simulink model "Simulador_CIC2021_Matlab2021a"  (R2021a)
settings: Solver=FixedStepAuto  StartTime=0.0  StopTime=inf  FixedStep=Ts  MaxStep=Ts  RelTol=1e-3
InitFcn:
  | Ts_com =0.0200;
  | Ts= 0.0100;
  | load DatosCref;
StopFcn:
  | clear tf Ts Ts_com tout DatosCrefC1 DatosCrefC2;
undefined symbols (not defined in the file): sigbuilder_block, Ts3
settings Model: Creator=jarico  LastModifiedBy=javier
settings SolverCC: ZeroCrossControl=DisableAll  AlgebraicLoopSolver=TrustRegion
settings DataIOCC: SaveFormat=StructureWithTime  SignalLogging=off  DSMLogging=off  ReturnWorkspaceOutputs=off
settings DebuggingCC: SFMachineParentedDataDiag=warning  ArithmeticOperatorsInVariantConditions=warning
settings SFSimCC: CustomCodeUndefinedFunction=UseInterfaceOnly

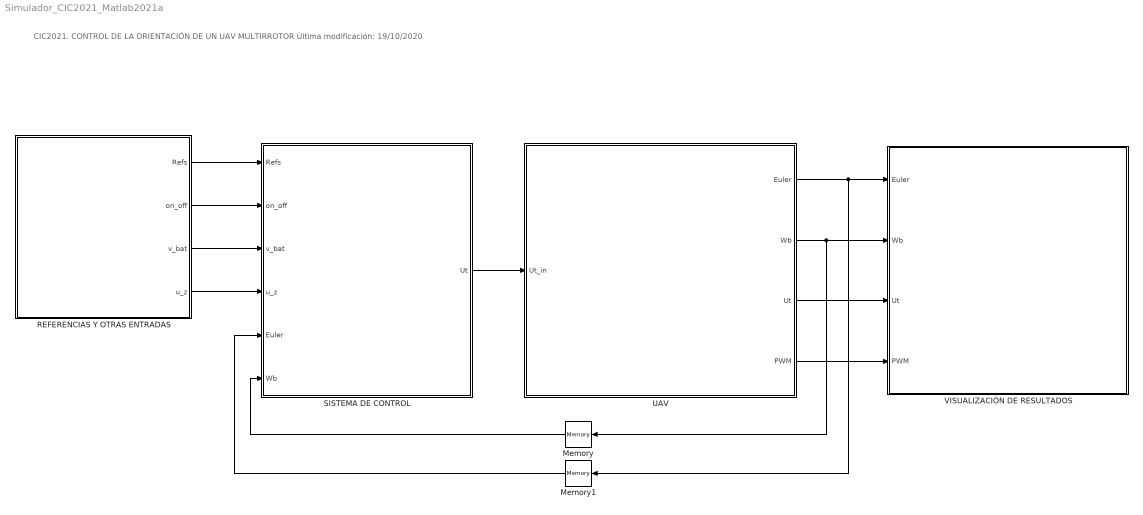
== system Simulador_CIC2021_Matlab2021a ==
  note: CIC2021. CONTROL DE LA ORIENTACIÓN DE UN UAV MULTIRROTOR
      |
      | Última modificación: 19/10/2020
  Memory : Memory
  Memory1 : Memory
  REFERENCIAS Y OTRAS ENTRADAS : Subsystem
  SISTEMA DE CONTROL : Subsystem
  UAV : Subsystem  SystemSampleTime=Ts3  mask(CONCURSO DE INGENIERÍA DE CONTROL CIC2021){Categoria=Categoría 1}
      mask prompts: Categoria "Seleccione categoría:"
      mask help: Modelo dinámico del UAV
      mask TypeOptions Categoria: Categoría 1 | Categoría 2
      mask DialogControl Container7 Prompt: Operación del sistema
      mask Display: image(imread('UAV.png'));
  VISUALIZACIÓN DE RESULTADOS : Subsystem
  wires:
  UAV/4(PWM) -> VISUALIZACIÓN DE RESULTADOS/4(PWM)
  UAV/3(Ut) -> VISUALIZACIÓN DE RESULTADOS/3(Ut)
  REFERENCIAS Y OTRAS ENTRADAS/1(Refs) -> SISTEMA DE CONTROL/1(Refs)
  REFERENCIAS Y OTRAS ENTRADAS/2(on_off) -> SISTEMA DE CONTROL/2(on_off)
  REFERENCIAS Y OTRAS ENTRADAS/3(v_bat) -> SISTEMA DE CONTROL/3(v_bat)
  REFERENCIAS Y OTRAS ENTRADAS/4(u_z) -> SISTEMA DE CONTROL/4(u_z)
  SISTEMA DE CONTROL/1(Ut) -> UAV/1(Ut_in)
  UAV/2(Wb) -> Memory/1, VISUALIZACIÓN DE RESULTADOS/2(Wb)
  UAV/1(Euler) -> Memory1/1, VISUALIZACIÓN DE RESULTADOS/1(Euler)
  Memory/1 -> SISTEMA DE CONTROL/6(Wb)
  Memory1/1 -> SISTEMA DE CONTROL/5(Euler)

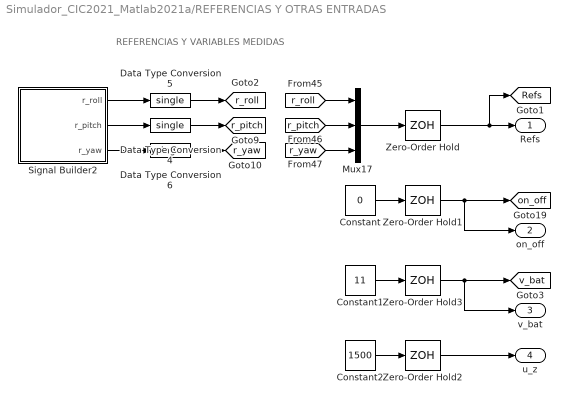
== system Simulador_CIC2021_Matlab2021a/REFERENCIAS Y OTRAS ENTRADAS ==
  note: REFERENCIAS Y VARIABLES MEDIDAS
  Constant : Constant  Value=0  OutDataTypeStr=int16
  Constant1 : Constant  Value=11  OutDataTypeStr=single
  Constant2 : Constant  Value=1500  OutDataTypeStr=single
  Data Type Conversion4 : DataTypeConversion  OutDataTypeStr=single
  Data Type Conversion5 : DataTypeConversion  OutDataTypeStr=single
  Data Type Conversion6 : DataTypeConversion  OutDataTypeStr=single
  Mux17 : Mux  Inputs=3
  Signal Builder2 : Subsystem  Tag=STV Subsys  LoadFcn=sigbuilder_block('load');  StartFcn=sigbuilder_block('start');  StopFcn=sigbuilder_block('stop');  ClipboardFcn=sigbuilder_block('clipboard');  mask(Sigbuilder block){tuvar=[0:10]}
      mask help: Simulink:masks:SigbuilderBlock_MD
      mask init:
      | if ~strcmp(get_param(bdroot(gcbh),'SimulationStatus'),'stopped') tuvar = sigbuilder_block('maskInit'); end
      settings: CopyFcn=sigbuilder_block('copy');  DeleteFcn=sigbuilder_block('delete');  ModelCloseFcn=sigbuilder_block('modelClose');  PreSaveFcn=sigbuilder_block('preSave');  PauseFcn=sigbuilder_block('pause');  ContinueFcn=sigbuilder_block('continue');  NameChangeFcn=sigbuilder_block('namechange');  OpenFcn=sigbuilder_block('open',[571.8 30.6 574.8 516.6 ]);  CloseFcn=sigbuilder_block('close');
      mask Display: plot(0, 0, 100, 100,[2, 2, 32, 32, 2], [68, 8, 8, 68, 68],[32, 2], [38, 38], [32, 19, 2],[53, 60, 44], [32, 17, 17, 2],[16, 16, 31, 31]);txt = getActiveGroup(gcbh);text(2, 100, txt,'verticalAlignment', 'top');
  Zero-Order Hold : ZeroOrderHold  SampleTime=Ts_com
  Zero-Order Hold1 : ZeroOrderHold  SampleTime=Ts_com
  Zero-Order Hold2 : ZeroOrderHold  SampleTime=Ts_com
  Zero-Order Hold3 : ZeroOrderHold  SampleTime=Ts
  Refs : Outport  VectorParamsAs1DForOutWhenUnconnected=off
  on_off : Outport  Port=2  VectorParamsAs1DForOutWhenUnconnected=off
  v_bat : Outport  Port=3  VectorParamsAs1DForOutWhenUnconnected=off
  u_z : Outport  Port=4  VectorParamsAs1DForOutWhenUnconnected=off
  tag scope: Refs=global, on_off=global, r_pitch=global, r_roll=global, r_yaw=global, v_bat=global
  wires:
  Constant/1 -> Zero-Order Hold1/1
  Mux17/1 -> Zero-Order Hold/1
  [r_roll] -> Mux17/1
  Data Type Conversion5/1 -> [r_roll]
  Data Type Conversion6/1 -> [r_yaw]
  [r_pitch] -> Mux17/2
  Data Type Conversion4/1 -> [r_pitch]
  [r_yaw] -> Mux17/3
  Signal Builder2/3(r_yaw) -> Data Type Conversion6/1
  Signal Builder2/2(r_pitch) -> Data Type Conversion4/1
  Signal Builder2/1(r_roll) -> Data Type Conversion5/1
  Constant1/1 -> Zero-Order Hold3/1
  Constant2/1 -> Zero-Order Hold2/1
  Zero-Order Hold/1 -> [Refs], Refs/1
  Zero-Order Hold1/1 -> on_off/1, [on_off]
  Zero-Order Hold2/1 -> u_z/1
  Zero-Order Hold3/1 -> [v_bat], v_bat/1

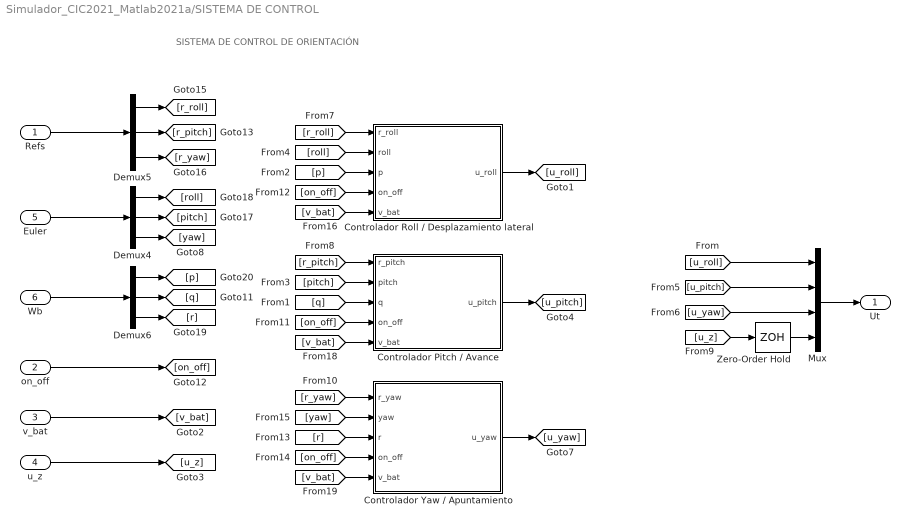
== system Simulador_CIC2021_Matlab2021a/SISTEMA DE CONTROL ==
  note: SISTEMA DE CONTROL DE ORIENTACIÓN
  Refs : Inport
  on_off : Inport  Port=2
  v_bat : Inport  Port=3
  u_z : Inport  Port=4
  Euler : Inport  Port=5
  Wb : Inport  Port=6
  Controlador Pitch / Avance : Subsystem
  Controlador Roll / Desplazamiento lateral : Subsystem
  Controlador Yaw / Apuntamiento : Subsystem
  Demux4 : Demux  Outputs=3
  Demux5 : Demux  Outputs=3
  Demux6 : Demux  Outputs=3
  Mux : Mux
  Zero-Order Hold : ZeroOrderHold  SampleTime=Ts
  Ut : Outport  VectorParamsAs1DForOutWhenUnconnected=off
  wires:
  [p] -> Controlador Roll / Desplazamiento lateral/3(p)
  [roll] -> Controlador Roll / Desplazamiento lateral/2(roll)
  [r_roll] -> Controlador Roll / Desplazamiento lateral/1(r_roll)
  Controlador Pitch / Avance/1(u_pitch) -> [u_pitch]
  Controlador Roll / Desplazamiento lateral/1(u_roll) -> [u_roll]
  [on_off] -> Controlador Roll / Desplazamiento lateral/4(on_off)
  [r_pitch] -> Controlador Pitch / Avance/1(r_pitch)
  [pitch] -> Controlador Pitch / Avance/2(pitch)
  [q] -> Controlador Pitch / Avance/3(q)
  [on_off] -> Controlador Pitch / Avance/4(on_off)
  [u_roll] -> Mux/1
  [u_pitch] -> Mux/2
  [u_yaw] -> Mux/3
  [u_z] -> Zero-Order Hold/1
  Mux/1 -> Ut/1
  Demux5/1 -> [r_roll]
  Demux4/2 -> [pitch]
  Demux4/3 -> [yaw]
  Demux5/2 -> [r_pitch]
  Demux5/3 -> [r_yaw]
  Demux4/1 -> [roll]
  Demux6/2 -> [q]
  Wb/1 -> Demux6/1
  Demux6/1 -> [p]
  Refs/1 -> Demux5/1
  on_off/1 -> [on_off]
  Euler/1 -> Demux4/1
  Demux6/3 -> [r]
  u_z/1 -> [u_z]
  v_bat/1 -> [v_bat]
  [yaw] -> Controlador Yaw / Apuntamiento/2(yaw)
  Controlador Yaw / Apuntamiento/1(u_yaw) -> [u_yaw]
  [on_off] -> Controlador Yaw / Apuntamiento/4(on_off)
  [r] -> Controlador Yaw / Apuntamiento/3(r)
  [r_yaw] -> Controlador Yaw / Apuntamiento/1(r_yaw)
  [v_bat] -> Controlador Roll / Desplazamiento lateral/5(v_bat)
  [v_bat] -> Controlador Pitch / Avance/5(v_bat)
  [v_bat] -> Controlador Yaw / Apuntamiento/5(v_bat)
  Zero-Order Hold/1 -> Mux/4

== system Simulador_CIC2021_Matlab2021a/UAV ==
  Ut_in : Inport
  " UAV" : Subsystem
      mask help: Simulink:masks:GenSFuncDesc_MD
      mask Help: eval('feval(''rtwprivate'',''rtwhelpview'',''rtw_sfcn_block'')');
  Constant : Constant  Value=Categoria
  Data Type Conversion : DataTypeConversion  OutDataTypeStr=single
  Demux : Demux
  Euler : Outport  VectorParamsAs1DForOutWhenUnconnected=off
  Wb : Outport  Port=2  VectorParamsAs1DForOutWhenUnconnected=off
  Ut : Outport  Port=3  VectorParamsAs1DForOutWhenUnconnected=off
  PWM : Outport  Port=4  VectorParamsAs1DForOutWhenUnconnected=off
  tag scope: Categoria=global
  wires:
  Demux/4 -> " UAV"/4(u_z)
  [v_bat] -> " UAV"/5(v_bat)
  Constant/1 -> Data Type Conversion/1
  " UAV"/3(Ut) -> Ut/1
  " UAV"/4(PWM) -> PWM/1
  " UAV"/1(Euler) -> Euler/1
  " UAV"/2(Wb) -> Wb/1
  Demux/3 -> " UAV"/3(u_yaw)
  Demux/2 -> " UAV"/2(u_pitch)
  Demux/1 -> " UAV"/1(u_roll)
  Ut_in/1 -> Demux/1
  Data Type Conversion/1 -> " UAV"/6(Categoria), [Categoria]

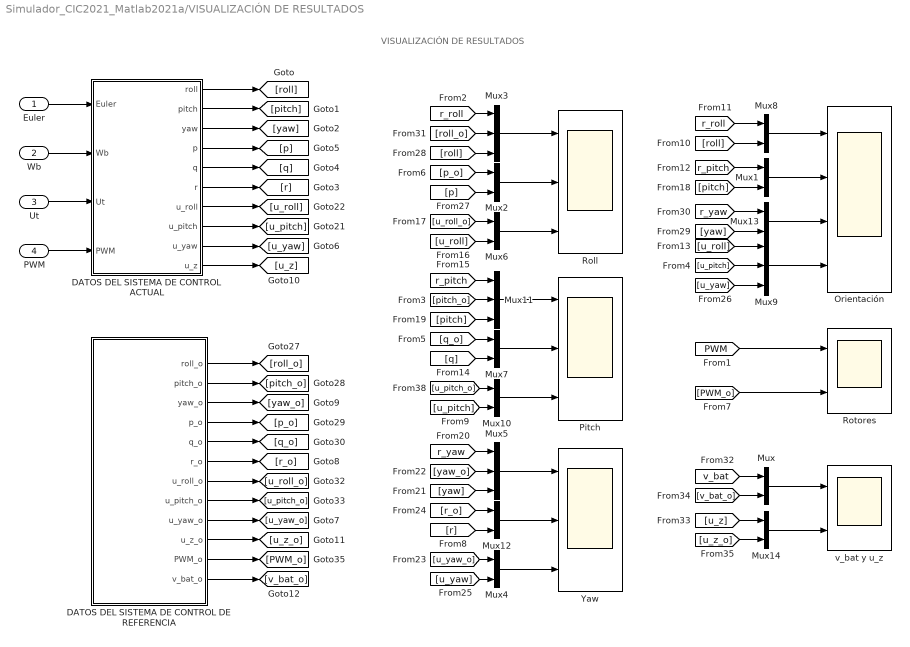
== system Simulador_CIC2021_Matlab2021a/VISUALIZACIÓN DE RESULTADOS ==
  note: VISUALIZACIÓN DE RESULTADOS
  Euler : Inport
  Wb : Inport  Port=2
  Ut : Inport  Port=3
  PWM : Inport  Port=4
  DATOS DEL SISTEMA DE CONTROL ACTUAL : Subsystem
  DATOS DEL SISTEMA DE CONTROL DE REFERENCIA : Subsystem
  Mux{,1..2,4,6..8,10,12..14} (11 alike) : Mux  Inputs=2
  Mux{3,5,9,11} (4 alike) : Mux  Inputs=3
  Orientación : Scope  NumInputPorts=4
  Pitch : Scope  NumInputPorts=3
  Roll : Scope  NumInputPorts=3
  Rotores : Scope  NumInputPorts=2
  Yaw : Scope  NumInputPorts=3
  v_bat y u_z : Scope  NumInputPorts=2
  wires:
  DATOS DEL SISTEMA DE CONTROL DE REFERENCIA/9(u_yaw_o) -> [u_yaw_o]
  DATOS DEL SISTEMA DE CONTROL DE REFERENCIA/6(r_o) -> [r_o]
  DATOS DEL SISTEMA DE CONTROL DE REFERENCIA/3(yaw_o) -> [yaw_o]
  DATOS DEL SISTEMA DE CONTROL ACTUAL/9(u_yaw) -> [u_yaw]
  DATOS DEL SISTEMA DE CONTROL ACTUAL/6(r) -> [r]
  DATOS DEL SISTEMA DE CONTROL ACTUAL/3(yaw) -> [yaw]
  [yaw] -> Mux13/2
  [r_yaw] -> Mux13/1
  Mux13/1 -> Orientación/3
  [u_yaw] -> Mux9/3
  [r_o] -> Mux12/1
  [u_yaw_o] -> Mux4/1
  [yaw] -> Mux5/3
  [yaw_o] -> Mux5/2
  [u_yaw] -> Mux4/2
  [r] -> Mux12/2
  [r_yaw] -> Mux5/1
  Mux4/1 -> Yaw/3
  Mux12/1 -> Yaw/2
  Mux5/1 -> Yaw/1
  Mux11/1 -> Pitch/1
  Mux7/1 -> Pitch/2
  Mux10/1 -> Pitch/3
  [r_pitch] -> Mux11/1
  [q] -> Mux7/2
  [u_pitch] -> Mux10/2
  Mux6/1 -> Roll/3
  Mux2/1 -> Roll/2
  [u_roll] -> Mux6/2
  [p] -> Mux2/2
  PWM/1 -> DATOS DEL SISTEMA DE CONTROL ACTUAL/4(PWM)
  DATOS DEL SISTEMA DE CONTROL ACTUAL/8(u_pitch) -> [u_pitch]
  DATOS DEL SISTEMA DE CONTROL ACTUAL/7(u_roll) -> [u_roll]
  DATOS DEL SISTEMA DE CONTROL ACTUAL/5(q) -> [q]
  DATOS DEL SISTEMA DE CONTROL ACTUAL/4(p) -> [p]
  DATOS DEL SISTEMA DE CONTROL ACTUAL/2(pitch) -> [pitch]
  DATOS DEL SISTEMA DE CONTROL ACTUAL/1(roll) -> [roll]
  Ut/1 -> DATOS DEL SISTEMA DE CONTROL ACTUAL/3(Ut)
  Wb/1 -> DATOS DEL SISTEMA DE CONTROL ACTUAL/2(Wb)
  Euler/1 -> DATOS DEL SISTEMA DE CONTROL ACTUAL/1(Euler)
  DATOS DEL SISTEMA DE CONTROL DE REFERENCIA/4(p_o) -> [p_o]
  DATOS DEL SISTEMA DE CONTROL DE REFERENCIA/5(q_o) -> [q_o]
  DATOS DEL SISTEMA DE CONTROL DE REFERENCIA/11(PWM_o) -> [PWM_o]
  DATOS DEL SISTEMA DE CONTROL DE REFERENCIA/7(u_roll_o) -> [u_roll_o]
  DATOS DEL SISTEMA DE CONTROL DE REFERENCIA/8(u_pitch_o) -> [u_pitch_o]
  DATOS DEL SISTEMA DE CONTROL DE REFERENCIA/1(roll_o) -> [roll_o]
  DATOS DEL SISTEMA DE CONTROL DE REFERENCIA/2(pitch_o) -> [pitch_o]
  [PWM] -> Rotores/1
  [pitch_o] -> Mux11/2
  [pitch] -> Mux11/3
  [r_roll] -> Mux3/1
  Mux9/1 -> Orientación/4
  [u_pitch_o] -> Mux10/1
  [q_o] -> Mux7/1
  [p_o] -> Mux2/1
  [u_roll_o] -> Mux6/1
  Mux3/1 -> Roll/1
  Mux1/1 -> Orientación/2
  [u_pitch] -> Mux9/2
  [u_roll] -> Mux9/1
  [pitch] -> Mux1/2
  [r_pitch] -> Mux1/1
  Mux8/1 -> Orientación/1
  [r_roll] -> Mux8/1
  [roll] -> Mux8/2
  [roll_o] -> Mux3/2
  [roll] -> Mux3/3
  [PWM_o] -> Rotores/2
  DATOS DEL SISTEMA DE CONTROL ACTUAL/10(u_z) -> [u_z]
  [v_bat] -> Mux/1
  [u_z] -> Mux14/1
  DATOS DEL SISTEMA DE CONTROL DE REFERENCIA/10(u_z_o) -> [u_z_o]
  DATOS DEL SISTEMA DE CONTROL DE REFERENCIA/12(v_bat_o) -> [v_bat_o]
  [v_bat_o] -> Mux/2
  [u_z_o] -> Mux14/2
  Mux/1 -> v_bat y u_z/1
  Mux14/1 -> v_bat y u_z/2

== system Simulador_CIC2021_Matlab2021a/REFERENCIAS Y OTRAS ENTRADAS/Signal Builder2 ==
  Demux : Demux  Tag=STV Demux  Outputs=3
      settings: DisplayOption=none
  FromWs : FromWorkspace  Tag=STV FromWs  VariableName=tuvar
      SigBuilderData=|
      | common.afterFinalStr = 'Extrapolate'
      | common.sampleTime = 0
      | dataSet.timeRange = [0 65]
      | dataSet.name = 'Group 1'
      | sbobj.Groups.Name = 'Group 1'
      | sbobj.Groups.Signals(1).Name = 'r_roll'
      | sbobj.Groups.Signals(1).XData = [0 5 5 10 10 25 25 30 30 40 40 65]
      | sbobj.Groups.Signals(1).YData = [0 0 200 200 0 0 -200 -200 200 200 0 0]
      | sbobj.Groups.Signals(2).Name = 'r_pitch'
      | sbobj.Groups.Signals(2).XData = [0 15 15 20 20 25 25 35 35 65]
      | sbobj.Groups.Signals(2).YData = [0 0 200 200 0 0 -200 -200 0 0]
      | sbobj.Groups.Signals(3).Name = 'r_yaw'
      | sbobj.Groups.Signals(3).XData = [0 45.3 50 55 60 65]
      | sbobj.Groups.Signals(3).YData = [0 0 -500 -500 0 0]
      | sbobj.Groups.TimeRange = [0 65]
  r_roll : Outport  Tag=STV Outport  VectorParamsAs1DForOutWhenUnconnected=off
  r_pitch : Outport  Tag=STV Outport  Port=2  VectorParamsAs1DForOutWhenUnconnected=off
  r_yaw : Outport  Tag=STV Outport  Port=3  VectorParamsAs1DForOutWhenUnconnected=off
  wires:
  Demux/3 -> r_yaw/1
  Demux/2 -> r_pitch/1
  FromWs/1 -> Demux/1
  Demux/1 -> r_roll/1

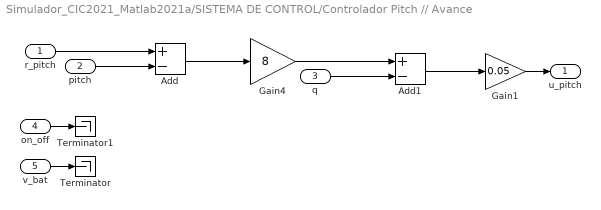
== system Simulador_CIC2021_Matlab2021a/SISTEMA DE CONTROL/Controlador Pitch // Avance ==
  r_pitch : Inport
  pitch : Inport  Port=2
  q : Inport  Port=3
  on_off : Inport  Port=4
  v_bat : Inport  Port=5
  Add : Sum  Inputs=+-
  Add1 : Sum  Inputs=+-
  Gain1 : Gain  Gain=0.05  OutDataTypeStr=single
  Gain4 : Gain  Gain=8
  Terminator : Terminator
  Terminator1 : Terminator
  u_pitch : Outport  VectorParamsAs1DForOutWhenUnconnected=off
  wires:
  Gain4/1 -> Add1/1
  r_pitch/1 -> Add/1
  Add/1 -> Gain4/1
  Add1/1 -> Gain1/1
  Gain1/1 -> u_pitch/1
  v_bat/1 -> Terminator/1
  on_off/1 -> Terminator1/1
  pitch/1 -> Add/2
  q/1 -> Add1/2

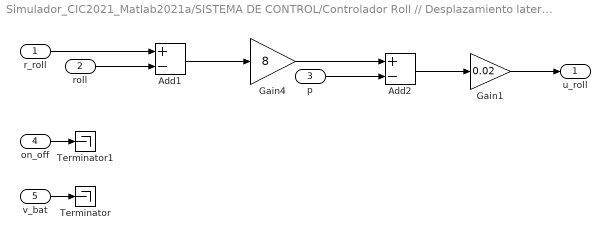
== system Simulador_CIC2021_Matlab2021a/SISTEMA DE CONTROL/Controlador Roll // Desplazamiento lateral ==
  r_roll : Inport
  roll : Inport  Port=2
  p : Inport  Port=3
  on_off : Inport  Port=4
  v_bat : Inport  Port=5
  Add1 : Sum  Inputs=+-
  Add2 : Sum  Inputs=+-
  Gain1 : Gain  Gain=0.02  OutDataTypeStr=single
  Gain4 : Gain  Gain=8
  Terminator : Terminator
  Terminator1 : Terminator
  u_roll : Outport  VectorParamsAs1DForOutWhenUnconnected=off
  wires:
  Gain1/1 -> u_roll/1
  v_bat/1 -> Terminator/1
  Gain4/1 -> Add2/1
  Add2/1 -> Gain1/1
  on_off/1 -> Terminator1/1
  Add1/1 -> Gain4/1
  r_roll/1 -> Add1/1
  roll/1 -> Add1/2
  p/1 -> Add2/2

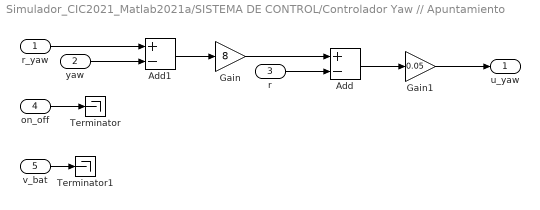
== system Simulador_CIC2021_Matlab2021a/SISTEMA DE CONTROL/Controlador Yaw // Apuntamiento ==
  r_yaw : Inport
  yaw : Inport  Port=2
  r : Inport  Port=3
  on_off : Inport  Port=4
  v_bat : Inport  Port=5
  Add : Sum  Inputs=+-
  Add1 : Sum  Inputs=+-
  Gain : Gain  Gain=8
  Gain1 : Gain  Gain=0.05
  Terminator : Terminator
  Terminator1 : Terminator
  u_yaw : Outport  VectorParamsAs1DForOutWhenUnconnected=off
  wires:
  r_yaw/1 -> Add1/1
  Add/1 -> Gain1/1
  Gain/1 -> Add/1
  r/1 -> Add/2
  yaw/1 -> Add1/2
  on_off/1 -> Terminator/1
  Add1/1 -> Gain/1
  Gain1/1 -> u_yaw/1
  v_bat/1 -> Terminator1/1

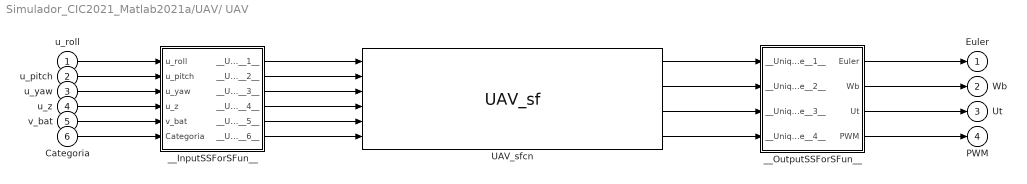
== system Simulador_CIC2021_Matlab2021a/UAV/ UAV ==
  u_roll : Inport
  u_pitch : Inport  Port=2
  u_yaw : Inport  Port=3
  u_z : Inport  Port=4
  v_bat : Inport  Port=5
  Categoria : Inport  Port=6
  " UAV_sfcn" : S-Function  FunctionName=UAV_sf  SFunctionModules=""  SFunctionDeploymentMode=off  EnableBusSupport=off  SFcnStateName=DWORK0  mask{rtw_sf_name=UAV_sf, showVar=off}
      mask prompts: rtw_sf_name "Simulink:masks:GenSFuncName_MP"; showVar "Simulink:masks:GenSFuncShowModuleList_MP"
      mask help: Simulink:masks:GenSFuncDesc_MD
      mask init:
      | displist = '';
      | if ~strcmp(get_param(gcb, 'FunctionName'), rtw_sf_name);
      |   set_param(gcb, 'FunctionName', rtw_sf_name);
      | end
      | % Check if we are generating code
      | rtw_mode = false;
      | if strcmpi(get_param(bdroot(gcb),'SimulationStatus'),'Initializing')
      | 	rtw_mode = strcmpi(get_param(bdroot(gcb),'BuildingRTWCode'),'on') && ...
      | 		~strcmpi(get_param(bdroot(gcb),'TargetStyle'),'SimulationTarget');
      | end
      | if showVar || rtw_mode
      | 	if exist('rtwsfunc') == 2 | exist('rtwsfunc') == 6
      | 		tmplist = rtwsfunc(rtw_sf_name,gcb);
      | 		tmplist = DAStudio.message('Simulink:masks:GenSFuncListOfModules_IC', tmplist);
      | 	elseif showVar
      | 		tmplist1 = DAStudio.message('Simulink:masks:GenSFuncListOfModules_IC', '');
      |         tmplist2 = DAStudio.message('Simulink:masks:GenSFuncNotLicensed_IC');
      |         tmplist = [tmplist1 tmplist2];
      |  	end
      | end
      | if showVar
      |   displist = tmplist;
      | end
      settings: SFcnIsStateOwnerBlock=on
      settings: CopyFcn=|
      | if ~strcmp(get_param(gcb,'Linkstatus'),'none') && ...
      | ~strcmp(get_param(gcb,'Linkstatus'),'implicit')
      |   set_param(gcb,'LinkStatus','none');
      | end
      mask Help: eval('feval(''rtwprivate'',''rtwhelpview'',''rtw_sfcn_block'')');
      mask Display:
      | port_label('input',1,'u_roll');
      | port_label('input',2,'u_pitch');
      | port_label('input',3,'u_yaw');
      | port_label('input',4,'u_z');
      | port_label('input',5,'v_bat');
      | port_label('input',6,'Categoria');
      | port_label('output',1,'Euler');
      | port_label('output',2,'Wb');
      | port_label('output',3,'Ut');
      | port_label('output',4,'PWM');
  __InputSSForSFun__ : Subsystem
  __OutputSSForSFun__ : Subsystem
  Euler : Outport  VectorParamsAs1DForOutWhenUnconnected=off
  Wb : Outport  Port=2  VectorParamsAs1DForOutWhenUnconnected=off
  Ut : Outport  Port=3  VectorParamsAs1DForOutWhenUnconnected=off
  PWM : Outport  Port=4  VectorParamsAs1DForOutWhenUnconnected=off
  wires:
  u_roll/1 -> __InputSSForSFun__/1(u_roll)
  u_pitch/1 -> __InputSSForSFun__/2(u_pitch)
  u_yaw/1 -> __InputSSForSFun__/3(u_yaw)
  u_z/1 -> __InputSSForSFun__/4(u_z)
  v_bat/1 -> __InputSSForSFun__/5(v_bat)
  Categoria/1 -> __InputSSForSFun__/6(Categoria)
  __InputSSForSFun__/1(__UniqueOutportName__1__) -> " UAV_sfcn"/1
  __InputSSForSFun__/2(__UniqueOutportName__2__) -> " UAV_sfcn"/2
  __InputSSForSFun__/3(__UniqueOutportName__3__) -> " UAV_sfcn"/3
  __InputSSForSFun__/4(__UniqueOutportName__4__) -> " UAV_sfcn"/4
  __InputSSForSFun__/5(__UniqueOutportName__5__) -> " UAV_sfcn"/5
  __InputSSForSFun__/6(__UniqueOutportName__6__) -> " UAV_sfcn"/6
  " UAV_sfcn"/1 -> __OutputSSForSFun__/1(__UniqueInportName__1__)
  " UAV_sfcn"/2 -> __OutputSSForSFun__/2(__UniqueInportName__2__)
  " UAV_sfcn"/3 -> __OutputSSForSFun__/3(__UniqueInportName__3__)
  " UAV_sfcn"/4 -> __OutputSSForSFun__/4(__UniqueInportName__4__)
  __OutputSSForSFun__/1(Euler) -> Euler/1
  __OutputSSForSFun__/2(Wb) -> Wb/1
  __OutputSSForSFun__/3(Ut) -> Ut/1
  __OutputSSForSFun__/4(PWM) -> PWM/1

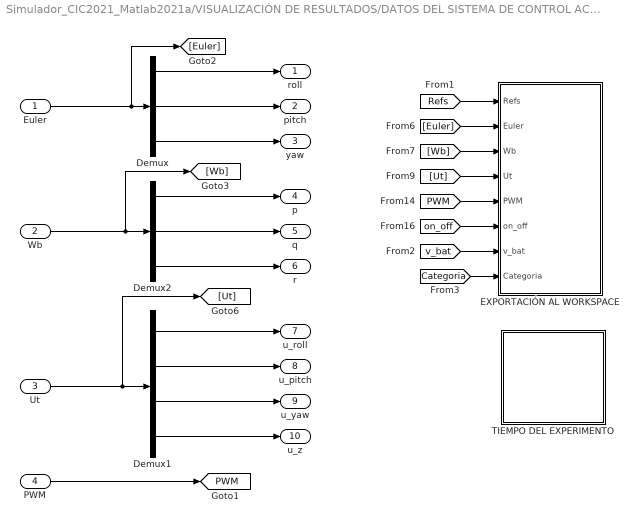
== system Simulador_CIC2021_Matlab2021a/VISUALIZACIÓN DE RESULTADOS/DATOS DEL SISTEMA DE CONTROL ACTUAL ==
  Euler : Inport
  Wb : Inport  Port=2
  Ut : Inport  Port=3
  PWM : Inport  Port=4
  Demux : Demux  Outputs=3
  Demux1 : Demux
  Demux2 : Demux  Outputs=3
  EXPORTACIÓN AL WORKSPACE : Subsystem
  TIEMPO DEL EXPERIMENTO : Subsystem
  roll : Outport  VectorParamsAs1DForOutWhenUnconnected=off
  pitch : Outport  Port=2  VectorParamsAs1DForOutWhenUnconnected=off
  yaw : Outport  Port=3  VectorParamsAs1DForOutWhenUnconnected=off
  p : Outport  Port=4  VectorParamsAs1DForOutWhenUnconnected=off
  q : Outport  Port=5  VectorParamsAs1DForOutWhenUnconnected=off
  r : Outport  Port=6  VectorParamsAs1DForOutWhenUnconnected=off
  u_roll : Outport  Port=7  VectorParamsAs1DForOutWhenUnconnected=off
  u_pitch : Outport  Port=8  VectorParamsAs1DForOutWhenUnconnected=off
  u_yaw : Outport  Port=9  VectorParamsAs1DForOutWhenUnconnected=off
  u_z : Outport  Port=10  VectorParamsAs1DForOutWhenUnconnected=off
  tag scope: PWM=global
  wires:
  PWM/1 -> [PWM]
  [Euler] -> EXPORTACIÓN AL WORKSPACE/2(Euler)
  [PWM] -> EXPORTACIÓN AL WORKSPACE/5(PWM)
  [Refs] -> EXPORTACIÓN AL WORKSPACE/1(Refs)
  [on_off] -> EXPORTACIÓN AL WORKSPACE/6(on_off)
  [Ut] -> EXPORTACIÓN AL WORKSPACE/4(Ut)
  [Wb] -> EXPORTACIÓN AL WORKSPACE/3(Wb)
  Demux2/1 -> p/1
  Demux2/2 -> q/1
  Demux1/2 -> u_pitch/1
  Demux/1 -> roll/1
  Demux/3 -> yaw/1
  Euler/1 -> Demux/1, [Euler]
  Demux2/3 -> r/1
  Demux1/1 -> u_roll/1
  Demux1/3 -> u_yaw/1
  Demux/2 -> pitch/1
  Wb/1 -> Demux2/1, [Wb]
  Ut/1 -> [Ut], Demux1/1
  Demux1/4 -> u_z/1
  [v_bat] -> EXPORTACIÓN AL WORKSPACE/7(v_bat)
  [Categoria] -> EXPORTACIÓN AL WORKSPACE/8(Categoria)

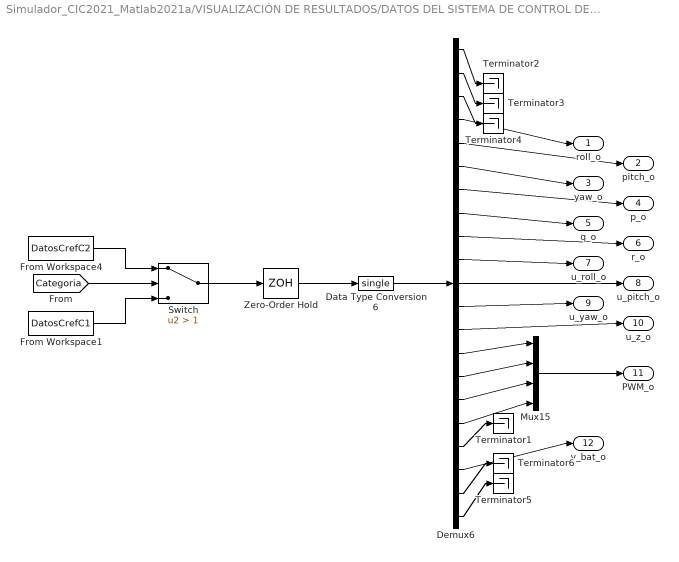
== system Simulador_CIC2021_Matlab2021a/VISUALIZACIÓN DE RESULTADOS/DATOS DEL SISTEMA DE CONTROL DE REFERENCIA ==
  Data Type Conversion6 : DataTypeConversion  OutDataTypeStr=single
  Demux6 : Demux  Outputs=21
  From Workspace1 : FromWorkspace  VariableName=DatosCrefC1
  From Workspace4 : FromWorkspace  VariableName=DatosCrefC2
  Mux15 : Mux
  Switch : Switch  Criteria=u2 > Threshold  Threshold=1
  Terminator{1..6} (6 alike) : Terminator
  Zero-Order Hold : ZeroOrderHold  SampleTime=Ts_com
  roll_o : Outport  VectorParamsAs1DForOutWhenUnconnected=off
  pitch_o : Outport  Port=2  VectorParamsAs1DForOutWhenUnconnected=off
  yaw_o : Outport  Port=3  VectorParamsAs1DForOutWhenUnconnected=off
  p_o : Outport  Port=4  VectorParamsAs1DForOutWhenUnconnected=off
  q_o : Outport  Port=5  VectorParamsAs1DForOutWhenUnconnected=off
  r_o : Outport  Port=6  VectorParamsAs1DForOutWhenUnconnected=off
  u_roll_o : Outport  Port=7  VectorParamsAs1DForOutWhenUnconnected=off
  u_pitch_o : Outport  Port=8  VectorParamsAs1DForOutWhenUnconnected=off
  u_yaw_o : Outport  Port=9  VectorParamsAs1DForOutWhenUnconnected=off
  u_z_o : Outport  Port=10  VectorParamsAs1DForOutWhenUnconnected=off
  PWM_o : Outport  Port=11  VectorParamsAs1DForOutWhenUnconnected=off
  v_bat_o : Outport  Port=12  VectorParamsAs1DForOutWhenUnconnected=off
  wires:
  Demux6/18 -> Terminator1/1
  Demux6/12 -> u_yaw_o/1
  Demux6/9 -> r_o/1
  Demux6/11 -> u_pitch_o/1
  Demux6/5 -> pitch_o/1
  Demux6/10 -> u_roll_o/1
  Mux15/1 -> PWM_o/1
  Demux6/7 -> p_o/1
  Demux6/8 -> q_o/1
  Demux6/4 -> roll_o/1
  From Workspace4/1 -> Switch/1
  Demux6/3 -> Terminator4/1
  Demux6/15 -> Mux15/2
  Demux6/17 -> Mux15/4
  Demux6/1 -> Terminator2/1
  Demux6/14 -> Mux15/1
  Data Type Conversion6/1 -> Demux6/1
  Demux6/6 -> yaw_o/1
  Demux6/2 -> Terminator3/1
  Demux6/16 -> Mux15/3
  Demux6/13 -> u_z_o/1
  Demux6/19 -> v_bat_o/1
  Demux6/20 -> Terminator6/1
  From Workspace1/1 -> Switch/3
  [Categoria] -> Switch/2
  Demux6/21 -> Terminator5/1
  Switch/1 -> Zero-Order Hold/1
  Zero-Order Hold/1 -> Data Type Conversion6/1

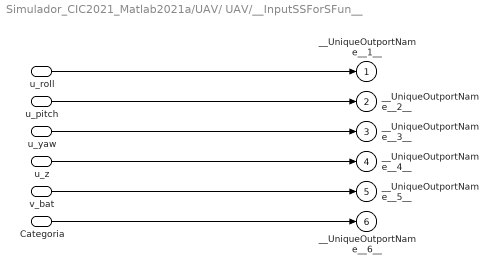
== system Simulador_CIC2021_Matlab2021a/UAV/ UAV/__InputSSForSFun__ ==
  u_roll : Inport
  u_pitch : Inport  Port=2
  u_yaw : Inport  Port=3
  u_z : Inport  Port=4
  v_bat : Inport  Port=5
  Categoria : Inport  Port=6
  __UniqueOutportName__1__ : Outport
  __UniqueOutportName__2__ : Outport  Port=2
  __UniqueOutportName__3__ : Outport  Port=3
  __UniqueOutportName__4__ : Outport  Port=4
  __UniqueOutportName__5__ : Outport  Port=5
  __UniqueOutportName__6__ : Outport  Port=6
  wires:
  u_roll/1 -> __UniqueOutportName__1__/1
  u_pitch/1 -> __UniqueOutportName__2__/1
  u_yaw/1 -> __UniqueOutportName__3__/1
  u_z/1 -> __UniqueOutportName__4__/1
  v_bat/1 -> __UniqueOutportName__5__/1
  Categoria/1 -> __UniqueOutportName__6__/1

== system Simulador_CIC2021_Matlab2021a/UAV/ UAV/__OutputSSForSFun__ ==
  __UniqueInportName__1__ : Inport
  __UniqueInportName__2__ : Inport  Port=2
  __UniqueInportName__3__ : Inport  Port=3
  __UniqueInportName__4__ : Inport  Port=4
  Euler : Outport  VectorParamsAs1DForOutWhenUnconnected=off
  Wb : Outport  Port=2  VectorParamsAs1DForOutWhenUnconnected=off
  Ut : Outport  Port=3  VectorParamsAs1DForOutWhenUnconnected=off
  PWM : Outport  Port=4  VectorParamsAs1DForOutWhenUnconnected=off
  wires:
  __UniqueInportName__1__/1 -> Euler/1
  __UniqueInportName__2__/1 -> Wb/1
  __UniqueInportName__3__/1 -> Ut/1
  __UniqueInportName__4__/1 -> PWM/1

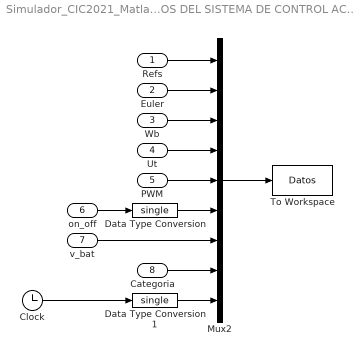
== system Simulador_CIC2021_Matlab2021a/VISUALIZACIÓN DE RESULTADOS/DATOS DEL SISTEMA DE CONTROL ACTUAL/EXPORTACIÓN AL WORKSPACE ==
  Refs : Inport
  Euler : Inport  Port=2
  Wb : Inport  Port=3
  Ut : Inport  Port=4
  PWM : Inport  Port=5
  on_off : Inport  Port=6
  v_bat : Inport  Port=7
  Categoria : Inport  Port=8
  Clock : Clock
  Data Type Conversion : DataTypeConversion  OutDataTypeStr=single
  Data Type Conversion1 : DataTypeConversion  OutDataTypeStr=single
  Mux2 : Mux  Inputs=9
  To Workspace : ToWorkspace  VariableName=Datos  SaveFormat=Structure With Time  SampleTime=-1
      settings: Decimation=2
  wires:
  PWM/1 -> Mux2/5
  Clock/1 -> Data Type Conversion1/1
  Refs/1 -> Mux2/1
  Mux2/1 -> To Workspace/1
  Euler/1 -> Mux2/2
  Wb/1 -> Mux2/3
  Data Type Conversion/1 -> Mux2/6
  on_off/1 -> Data Type Conversion/1
  Ut/1 -> Mux2/4
  v_bat/1 -> Mux2/7
  Data Type Conversion1/1 -> Mux2/9
  Categoria/1 -> Mux2/8

== system Simulador_CIC2021_Matlab2021a/VISUALIZACIÓN DE RESULTADOS/DATOS DEL SISTEMA DE CONTROL ACTUAL/TIEMPO DEL EXPERIMENTO ==
  Add : Sum  Inputs=+-
  Clock1 : Clock
  Constant : Constant  Value=65
  Constant1 : Constant  Value=45
  Constant2 : Constant  Value=0
  Constant3 : Constant
  Stop Simulation : Stop
  Switch1 : Switch  Criteria=u2 > Threshold  Threshold=1
  Switch2 : Switch
  wires:
  Constant3/1 -> Switch2/1
  Switch1/1 -> Add/2
  Constant/1 -> Switch1/1
  Constant2/1 -> Switch2/3
  Constant1/1 -> Switch1/3
  [Categoria] -> Switch1/2
  Add/1 -> Switch2/2
  Switch2/1 -> Stop Simulation/1
  Clock1/1 -> Add/1
